simulink model "seek_and_eat"  (R2016b)
settings: Solver=FixedStepAuto  StartTime=0.0  StopTime=10.0  RelTol=1e-3  EnableMultiTasking=on
libraries: legoev3lib x5
settings Model: ExtModeTrigDuration=2  Creator=Nexel  LastModifiedBy=Nexel
settings SolverCC: PositivePriorityOrder=on
settings OptimizationCC: MaxStackSize=64
settings DebuggingCC: ParameterTunabilityLossMsg=error
settings HardwareCC: ProdBitPerPointer=32  ProdBitPerSizeT=32  ProdBitPerPtrDiffT=32  ProdLargestAtomicInteger=Long  ProdWordSize=32  ProdHWDeviceType=ARM Compatible->ARM 9
settings RTWCC: SystemTargetFile=ert.tlc  HardwareBoard=LEGO MINDSTORMS EV3  TLCOptions="-aInlineSetEventsForThisBaseRateFcn=TLC_FALSE -aSuppressMultiTaskScheduler=TLC_FALSE  -aRateBasedStepFcn=0"  TemplateMakefile=ert_default_tmf  Description=Embedded Coder  GenerateReport=on  Toolchain=Sourcery G++ Lite v2009q3  IncludeHyperlinkInReport=on  LaunchReport=on  GenerateTraceInfo=on  GenerateTraceReport=on  GenerateTraceReportSl=on  GenerateTraceReportSf=on  GenerateTraceReportEml=on
settings CodeAppCC: ForceParamTrailComments=on  IgnoreCustomStorageClasses=off  OperatorAnnotations=on  SimulinkDataObjDesc=on  SFDataObjDesc=on  MATLABFcnDesc=on  InsertBlockDesc=on  MATLABSourceComments=on
settings ERTTargetCC: SupportContinuousTime=on  SupportVariableSizeSignals=on

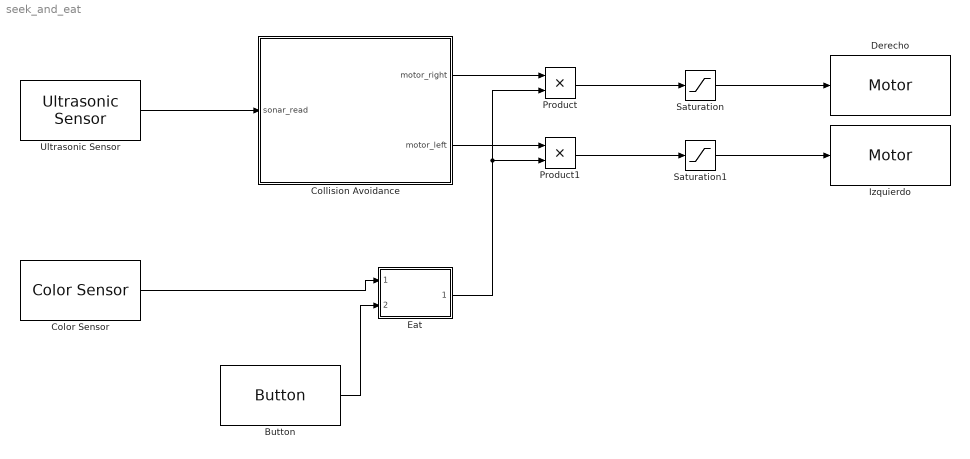
== system seek_and_eat ==
  Button : legoev3lib/Button  buttonType=Center  sampleTime=0.1
  Collision Avoidance : MATLAB Function  TreatAsAtomicUnit=on
  Color Sensor : legoev3lib/Color Sensor  portNumber=1  mode=Reflected light intensity  sampleTime=0.1
  Derecho : legoev3lib/Motor  sportNumber=D  sstopAction=Brake
  "Eat " : MATLAB Function  TreatAsAtomicUnit=on
  "Izquierdo " : legoev3lib/Motor  sportNumber=A  sstopAction=Brake
  Product : Product
  Product1 : Product
  Saturation : Saturate  UpperLimit=45  LowerLimit=-15
  Saturation1 : Saturate  UpperLimit=35  LowerLimit=-15
  Ultrasonic Sensor : legoev3lib/Ultrasonic Sensor  PortNumber=4  sampleTime=0.1
  wires:
  Ultrasonic Sensor/1 -> Collision Avoidance/1(sonar_read)
  Collision Avoidance/2(motor_left) -> Product1/1
  Collision Avoidance/1(motor_right) -> Product/1
  "Eat "/1(no_eating) -> Product1/2, Product/2
  Color Sensor/1 -> "Eat "/1(rgb_read)
  Button/1 -> "Eat "/2(button_pressed)
  Saturation1/1 -> "Izquierdo "/1
  Product1/1 -> Saturation1/1
  Product/1 -> Saturation/1
  Saturation/1 -> Derecho/1

== matlab function seek_and_eat/Eat  ==
  data: rgb_read input; no_eating output; button_pressed input
function no_eating  = eat(rgb_read, button_pressed)
    persistent no_eating_per
    if isempty(no_eating_per)
        no_eating_per = 1;
    end
    if (button_pressed == 1 && no_eating_per == 0)
        no_eating_per = 1;
    elseif(rgb_read > 60) 
        no_eating_per = 0;
    end
    no_eating = no_eating_per;

end

== matlab function seek_and_eat/Collision Avoidance ==
  data: sonar_read input; motor_right output; motor_left output
function [motor_right, motor_left] = fcn(sonar_read)
    if(sonar_read < 40 )
        motor_right = -50;
        motor_left = 50;
    else
        
        motor_right = round(100*rand);
        motor_left = round(100*rand);
    end
end
